simulink model "Sim_Second_Order_Consensus"  (R2020a)
settings: Solver=VariableStepAuto  StartTime=0.0  StopTime=10.0  RelTol=1e-6
values from neighbouring files (symbols this model uses):
  eta = input('Number of cycles eta : ')    [ComputeDWMGraphsJCF.m]    (also in ComputeDWMGraphsJCF_V1.m = eta; Dutchwindmill1010.mat = 10; Dutchwindmill22.mat = 2; Dutchwindmill23.mat = 2)
  Jtilde = inv(Phi_)*Ltilde*Phi_    [SecondOrderConsensusStateMatrixEigenSpace_V1.m]    (also in SecondOrderConsensusStateMatrixJCF.m)
  kappa = input('Number of nodes for each cycle kappa : ')    [ComputeDWMGraphsJCF.m]    (also in ComputeDWMGraphsJCF_V1.m = kappa; Dutchwindmill1010.mat = 10; Dutchwindmill22.mat = 2; Dutchwindmill23.mat = 3)
  L = D-A    [ComputeDWMGraphsJCF.m]    (also in ComputeDWMGraphsJCF_V1.m; Dutchwindmill1010.mat = [10 0 0 0 0 0 0 0 0 0 -1 0 ... (10201 elements, 101x101)]; Dutchwindmill22.mat = [2 0 -1 0 -1 -1 1 0 0 0 0 -1 ... (25 elements, 5x5)]; Dutchwindmill23.mat = [2 0 0 -1 0 0 -1 -1 1 0 0 0 ... (49 elements, 7x7)])
  Ltilde = [zeros(n,n),-eye(n);L xi*L]    [SecondOrderConsensusStateMatrixEigenSpace_V1.m]    (also in SecondOrderConsensusStateMatrixJCF.m)
  Phi_ = zeros(2*n,2*n)    [SecondOrderConsensusStateMatrixEigenSpace_V1.m]    (also in SecondOrderConsensusStateMatrixJCF.m)
  xi = ((mu1(i,j)+mu2(i,j))/(mu1(i,j)*mu2(i,j)))    [SecondOrderConsensusStateMatrixEigenSpace_V1.m]    (also in SecondOrderConsensusStateMatrixJCF.m = 1)
settings Model: Creator=francois.bateman  LastModifiedBy=francois.bateman
settings DataIOCC: ReturnWorkspaceOutputs=off

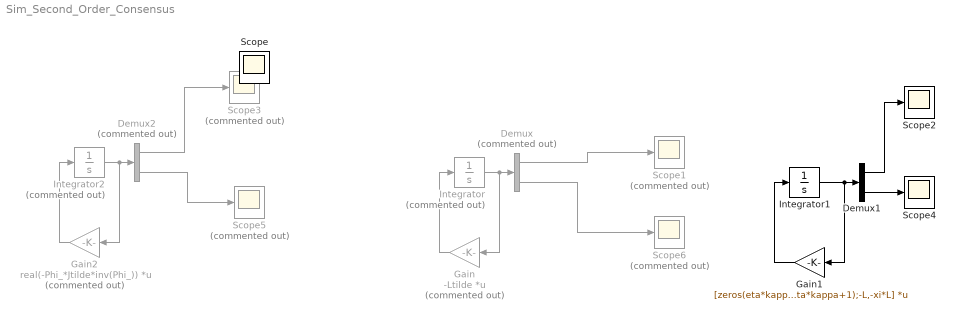
== system Sim_Second_Order_Consensus ==
  Demux : Demux  Commented=on  Outputs=[31,31]
  Demux1 : Demux  Outputs=[eta*kappa+1,eta*kappa+1]
  Demux2 : Demux  Commented=on  Outputs=[7,7]
  Gain : Gain  Commented=on  Gain=-Ltilde  Multiplication=Matrix(K*u)
  Gain1 : Gain  Gain=[zeros(eta*kappa+1),eye(eta*kappa+1);-L,-xi*L]  Multiplication=Matrix(K*u)
  Gain2 : Gain  Commented=on  Gain=real(-Phi_*Jtilde*inv(Phi_))  Multiplication=Matrix(K*u)
  Integrator : Integrator  Commented=on  InitialCondition=[randn((eta*kappa+1),1);zeros(eta*kappa+1,1) ]
  Integrator1 : Integrator  InitialCondition=[randn((eta*kappa+1),1);zeros(eta*kappa+1,1) ]
  Integrator2 : Integrator  Commented=on  InitialCondition=[randn((eta*kappa+1),1);zeros(eta*kappa+1,1) ]
  Scope{1,3,5..6} (4 alike) : Scope  Commented=on
  Scope2 : Scope
  Scope4 : Scope
  Scope : Scope
  wires:
  Gain/1 -> Integrator/1
  Integrator/1 -> Gain/1, Demux/1
  Demux/1 -> Scope1/1
  Demux1/1 -> Scope2/1
  Integrator1/1 -> Gain1/1, Demux1/1
  Gain1/1 -> Integrator1/1
  Demux2/1 -> Scope3/1
  Integrator2/1 -> Gain2/1, Demux2/1
  Gain2/1 -> Integrator2/1
  Demux1/2 -> Scope4/1
  Demux2/2 -> Scope5/1
  Demux/2 -> Scope6/1
